simulink model "fast_response"  (R2023b)
settings: Solver=VariableStepAuto  StartTime=0.0  StopTime=inf  RelTol=1e-3
libraries: audiosources x1, dspsnks4 x1, simulink x1
settings Model: Creator=Thinkpad  LastModifiedBy=Thinkpad

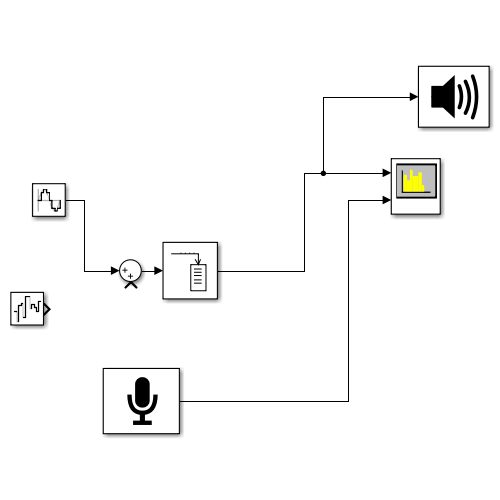
[thumbnail: Simulink's stored preview of the top-level diagram]
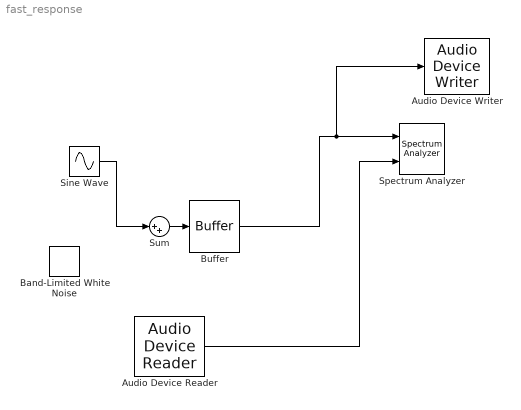
== system fast_response ==
  Audio Device Reader : audiosources/Audio Device Reader  Driver=DirectSound  Device=麦克风 (Scarlett 2i2 USB)  SampleRate=48000  NumChannels=2  SamplesPerFrame=1024  BitDepth=16-bit integer  NumBuffers=10  DefaultInputChannelMapping=on  InputChannelMapping=1:2  OutputNumOverrunSamples=off  OutputDataType=double  DriverIdx=1  DeviceWarnFlag=''
  Audio Device Writer : dspsnks4/Audio Device Writer  Driver=DirectSound  Device=扬声器 (Scarlett 2i2 USB)  InheritSampleRate=on  SampleRate=44100  BitDepth=16-bit integer  BufferSize=4096  NumBuffers=10  DefaultOutputChannelMapping=on  OutputChannelMapping=1:2  OutputNumUnderrunSamples=off  DriverIdx=1  DeviceWarnFlag=''
  Band-Limited White Noise : simulink/Sources/Band-Limited White Noise  Cov=[0.01]  Ts=1/48000  seed=[23341]
  Buffer : Buffer  N=1024  OutputFrames=off
  Sine Wave : Sin  Amplitude=10  Frequency=1000  SampleTime=1/48000
  Spectrum Analyzer : SpectrumAnalyzer  NumInputPorts=2  WindowPosition=[159.000000,87.000000,800.000000,500.000000,]  Visible=on  ScopeFrameLocation=window  SampleRateSource=Property  SampleRate=48000  PlotAsTwoSidedSpectrum=off  FrequencyScale=Log  FrequencySpan=Start and stop frequencies  StartFrequency=20  StopFrequency=20e3  RBW=2000  YLimits=[-119.46222278,65.4662365]
  Sum : Sum  Inputs=|++
  wires:
  Buffer/1 -> Audio Device Writer/1, Spectrum Analyzer/1
  Sine Wave/1 -> Sum/1
  Sum/1 -> Buffer/1
  Audio Device Reader/1 -> Spectrum Analyzer/2
